simulink model "exercise02_05"  (R2023b)
settings: Solver=VariableStepAuto  StartTime=0.0  StopTime=10.0  RelTol=1e-3
settings Model: Creator=aulas  LastModifiedBy=felip

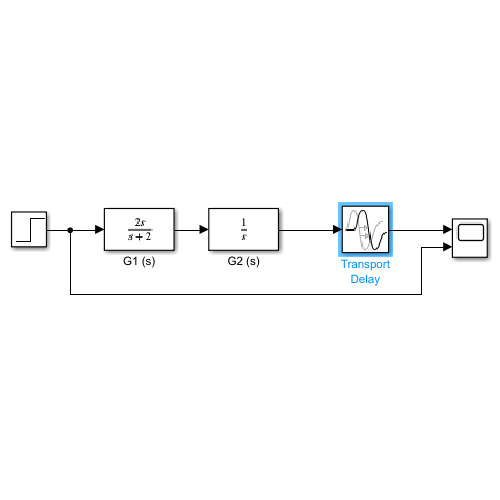
[thumbnail: Simulink's stored preview of the top-level diagram]
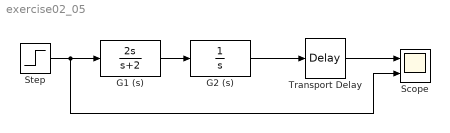
== system exercise02_05 ==
  G1 (s) : TransferFcn  Numerator=[2 0]  Denominator=[1 2]
  G2 (s) : TransferFcn  Denominator=[1 0]
  Scope : Scope  NumInputPorts=2
  Step : Step  SampleTime=0
  Transport Delay : TransportDelay  DelayTime=0.2
  wires:
  G1 (s)/1 -> G2 (s)/1
  G2 (s)/1 -> Transport Delay/1
  Transport Delay/1 -> Scope/1
  Step/1 -> Scope/2, G1 (s)/1
